simulink model "walkingRobotRL3D"  (R2020b)
settings: Solver=ode23t  StartTime=0.0  StopTime=Tf  RelTol=1e-2  EnableMultiTasking=on
PreLoadFcn:
  | robotParametersRL
undefined symbols (not defined in the file): agent, ankleD_pitch_jointMAX, ankleD_pitch_jointMIN, ankleD_roll_jointMAX, ankleD_roll_jointMIN, ankleI_pitch_jointMAX, ankleI_pitch_jointMIN, ankleI_roll_jointMAX, ankleI_roll_jointMIN, getSampleTime, height_plane, hipD_pitch_jointMAX, hipD_pitch_jointMIN, hipD_roll_jointMAX, hipD_roll_jointMIN, hipI_pitch_jointMAX, hipI_pitch_jointMIN, hipI_roll_jointMAX, hipI_roll_jointMIN, init_angs_L, init_angs_R, init_height, joint_damping, joint_limit_damping, joint_limit_stiffness, joint_stiffness, kneeD_jointMAX, kneeD_jointMIN, kneeI_jointMAX, kneeI_jointMIN, lower_leg_I0, lower_leg_length, lower_leg_mass, lower_leg_x, lower_leg_y, muscle_nominal_length, p10_ankleD_roll, plane_x, plane_y, regulator_type, tau, Tf, torso_height, torso_length, torso_offset_x, torso_offset_z, torso_width, torso_x, torso_y, torso_z, Ts, upper_leg_I0, upper_leg_length, upper_leg_mass, upper_leg_x, upper_leg_y, v10_ankleD_pitch, v10_ankleD_roll, v10_ankleI_pitch, v10_ankleI_roll ... (+41)
libraries: sm_lib x222, simulink x183, nesl_utility x130, walkingRobotUtils x69, rllib x2
(part 24 of 24)

== matlab function walkingRobotRL3D/Walking Robot (Angle based)/Antagonistic PAM Left Leg/ankleI_roll PAM/Proportional Regulator (Muscles 1) ==
  data: V1 input; reg_type input; p1 output
% Author: Eduardo Reyero Ibáñez
% Descrition: In this file it will be implemented the required input for the PAM
function p1  = propReg(V1,reg_type)
%% Proportional pressure regulators VPPM
%Range of Voltage
minVoltage = 0;
maxVoltage = 7.98; % This voltage provide 8 bar of pressure with regulator type 1
p1 = zeros(1,1);
%Select regulartor type
%reg_type = 1; % This will be given by the call of the function
%Limit the voltage
for i=1:length(p1)
if V1(i) >= maxVoltage 
    V1(i) = maxVoltage;
end
end
if reg_type == 1
    f_prop = @(V) 0.99*V+0.1;
    for i=1:length(p1)
    p1(i) = f_prop(V1(i));
    end
elseif reg_type == 2
    f_prop = @(V) 0.594*V+0.06;
    for i=1:length(p1)
    p1(i) = f_prop(V1(i));
    end
else
    f_prop = @(V) 0.198*V+0.02;
    for i=1:length(p1)
    p1(i) = f_prop(V1(i));
    end
end

% figure
% fplot(p1)
% xlim([0 10])
% ylim([0 10])
end

== matlab function walkingRobotRL3D/Walking Robot (Angle based)/Antagonistic PAM Left Leg/ankleI_roll PAM/Proportional Regulator (Muscles 2) ==
  data: V1 input; reg_type input; p1 output
% Author: Eduardo Reyero Ibáñez
% Descrition: In this file it will be implemented the required input for the PAM
function p1  = propReg(V1,reg_type)
%% Proportional pressure regulators VPPM
%Range of Voltage
minVoltage = 0;
maxVoltage = 7.98; % This voltage provide 8 bar of pressure with regulator type 1
p1 = zeros(1,1);
%Select regulartor type
%reg_type = 1; % This will be given by the call of the function
%Limit the voltage
for i=1:length(p1)
if V1(i) >= maxVoltage 
    V1(i) = maxVoltage;
end
end
if reg_type == 1
    f_prop = @(V) 0.99*V+0.1;
    for i=1:length(p1)
    p1(i) = f_prop(V1(i));
    end
elseif reg_type == 2
    f_prop = @(V) 0.594*V+0.06;
    for i=1:length(p1)
    p1(i) = f_prop(V1(i));
    end
else
    f_prop = @(V) 0.198*V+0.02;
    for i=1:length(p1)
    p1(i) = f_prop(V1(i));
    end
end

% figure
% fplot(p1)
% xlim([0 10])
% ylim([0 10])
end

== matlab function walkingRobotRL3D/Walking Robot (Angle based)/Antagonistic PAM Left Leg/ankleI_roll PAM/Spring and damping model/Stimation of spring coefficients ==
  data: P1 input; S1 output; Fload input; dmax1 input; F1 input; dmax1_per input
%Author: Eduardo Reyero
%Description: Calculate spring coefficient

function S1 = calculateSpringCoeff(P1,Fload,dmax1,F1,dmax1_per)
S1=zeros(length(dmax1),1);
%curve1 = @(x,P)  -0.002697-93.8*x+2.917*P+13.05*x^2-0.04264*x*P-0.001793*P^2-0.9395*x^3-0.001597*x^2*P-0.0001142*x*P^2+4.694e-06*P^3+0.03335*x^4+6.106e-06*x^3*P+2.699e-06*x^2*P^2+1.25e-07*x*P^3-5.675e-09*P^4-0.0004611*x^5+9.334e-07*x^4*P-1.221e-08*x^3*P^2-1.463e-09*x^2*P^3-4.929e-11*x*P^4+2.492e-12*P^5;
%F1 = zeros(length(P1),1);
for i=1:length(P1)
 %   F1(i) = curve1(dmax1_per(i),P1(i)); %Should be 0 (or aprox 0)
    S1(i) = (F1(i)-Fload(i))/dmax1(i); 
end
 
 %   S1(i) = 4379.43006090932;
end

== matlab function walkingRobotRL3D/Walking Robot (Angle based)/Antagonistic PAM Left Leg/ankleI_roll PAM/Spring and damping model/Stimation of spring coefficients1 ==
  data: F2 input; P2 input; S2 output; Fload input; dmax2 input; dmax2_per input
%Author: Eduardo Reyero
%Description: Calculate spring coefficient

function S2 = calculateSpringCoeff(F2,P2,Fload,dmax2,dmax2_per)
S2=zeros(length(dmax2),1);
%curve1 = @(x,P)  -0.002697-93.8*x+2.917*P+13.05*x^2-0.04264*x*P-0.001793*P^2-0.9395*x^3-0.001597*x^2*P-0.0001142*x*P^2+4.694e-06*P^3+0.03335*x^4+6.106e-06*x^3*P+2.699e-06*x^2*P^2+1.25e-07*x*P^3-5.675e-09*P^4-0.0004611*x^5+9.334e-07*x^4*P-1.221e-08*x^3*P^2-1.463e-09*x^2*P^3-4.929e-11*x*P^4+2.492e-12*P^5;
%F2 = zeros(length(P2),1);
for i=1:length(P2)
   % F2(i) = curve1(dmax2_per(i),P2(i)); %Should be aprox 0
    S2(i) = (F2(i)-Fload(i))/dmax2(i); 
end
  %  S2(i) = -8268.02654048148;
end

== matlab function walkingRobotRL3D/Walking Robot (Angle based)/Antagonistic PAM Left Leg/ankleI_roll PAM/Spring and damping model/getDeltaXmax/getMaxStroke1 ==
  data: P1 input; x_max1 output
%Author: Eduardo Reyero Ibáñez
%Description: Functions for obtaining the maximun stroke value of a given
%curve F(x). It is reached for the x value which makes F = 0
function x_max1 = getMaxStroke(P1)
x_range = (-3:0.01:29)'; %This range convers the %contraction for all the pressures from 0 to 8 bar
%load('StaticFxPmodel\fxpSurface.mat');

curve1 = @(x,P)  -0.002697-93.8*x+2.917*P+13.05*x^2-0.04264*x*P-0.001793*P^2-0.9395*x^3-0.001597*x^2*P-0.0001142*x*P^2+4.694e-06*P^3+0.03335*x^4+6.106e-06*x^3*P+2.699e-06*x^2*P^2+1.25e-07*x*P^3-5.675e-09*P^4-0.0004611*x^5+9.334e-07*x^4*P-1.221e-08*x^3*P^2-1.463e-09*x^2*P^3-4.929e-11*x*P^4+2.492e-12*P^5;
F_x = zeros(length(x_range),1);
for i=1:length(x_range)
    F_x(i) = curve1(x_range(i),P1);
    if F_x(i)<0
       %We have found the x axis cross
       x_max1 = x_range(i-1);
       break;
   else
        x_max1 = x_range(i); %Will never end here but need to avoid simulink error
    end
end

end

== matlab function walkingRobotRL3D/Walking Robot (Angle based)/Antagonistic PAM Left Leg/ankleI_roll PAM/Spring and damping model/getDeltaXmax1/getMaxStroke1 ==
  data: P2 input; x_max1 output
%Author: Eduardo Reyero Ibáñez
%Description: Functions for obtaining the maximun stroke value of a given
%curve F(x). It is reached for the x value which makes F = 0
function x_max1 = getMaxStroke(P2)
x_range = (-3:0.01:29)'; %This range convers the %contraction for all the pressures from 0 to 8 bar
%load('StaticFxPmodel\fxpSurface.mat');

curve1 = @(x,P)  -0.002697-93.8*x+2.917*P+13.05*x^2-0.04264*x*P-0.001793*P^2-0.9395*x^3-0.001597*x^2*P-0.0001142*x*P^2+4.694e-06*P^3+0.03335*x^4+6.106e-06*x^3*P+2.699e-06*x^2*P^2+1.25e-07*x*P^3-5.675e-09*P^4-0.0004611*x^5+9.334e-07*x^4*P-1.221e-08*x^3*P^2-1.463e-09*x^2*P^3-4.929e-11*x*P^4+2.492e-12*P^5;
F_x = zeros(length(x_range),1);
for i=1:length(x_range)
    F_x(i) = curve1(x_range(i),P2);
    if F_x(i)<0
       %We have found the x axis cross
       x_max1 = x_range(i-1);
       break;
   else
        x_max1 = x_range(i); %Will never end here but need to avoid simulink error
    end
end

end

== matlab function walkingRobotRL3D/Walking Robot1/Dynamic model of antagonistic PAM actuators/Spring//Damping (Muscles 1)/Getxmax1/getMaxStroke9 ==
  data: P1 input; x_max1 output
%Author: Eduardo Reyero Ibáñez
%Description: Functions for obtaining the maximun stroke value of a given
%curve F(x). It is reached for the x value which makes F = 0
function x_max1 = getMaxStroke(P1)
x_range = (-3:0.01:29)'; %This range convers the %contraction for all the pressures from 0 to 8 bar
%load('StaticFxPmodel\fxpSurface.mat');
curve1 = @(x,P)  -0.002697-93.8*x+2.917*P+13.05*x^2-0.04264*x*P-0.001793*P^2-0.9395*x^3-0.001597*x^2*P-0.0001142*x*P^2+4.694e-06*P^3+0.03335*x^4+6.106e-06*x^3*P+2.699e-06*x^2*P^2+1.25e-07*x*P^3-5.675e-09*P^4-0.0004611*x^5+9.334e-07*x^4*P-1.221e-08*x^3*P^2-1.463e-09*x^2*P^3-4.929e-11*x*P^4+2.492e-12*P^5;
F_x = zeros(length(x_range),1);
for i=1:length(x_range)
    F_x(i) = curve1(x_range(i),P1);
    if F_x(i)<0
       %We have found the x axis cross
       x_max1 = x_range(i-1);
       break;
   else
        x_max1 = x_range(i); %Will never end here but need to avoid simulink error
    end
end

end

== matlab function walkingRobotRL3D/Walking Robot (Angle based)/Antagonistic PAM Left Leg/ankleI_pitch PAM/F(x,P) mode (Muscles 1) ==
  data: P1 input; F1 output; x_muscle1 input
%Author: Eduardo Reyero Ibáñez
%Note: F(x) curves for different pressures are limited by recommended
%limitation of 20% in contraction percentage for the used PAM actuator
%(L = 260mm D=20mm)
function F1 = FxPmodel(P1,x_muscle1)
%Input: P comming from proporcional controller  is in bar. Its 6x1 vector
% x_muscle (in % contraction)
%Output:F according to P input and and x value of half of the maximun
%permissible stroke
%Importing 2 variable F(x,P) model
curve = @(x,P)  -0.002697-93.8*x+2.917*P+13.05*x^2-0.04264*x*P-0.001793*P^2-0.9395*x^3-0.001597*x^2*P-0.0001142*x*P^2+4.694e-06*P^3+0.03335*x^4+6.106e-06*x^3*P+2.699e-06*x^2*P^2+1.25e-07*x*P^3-5.675e-09*P^4-0.0004611*x^5+9.334e-07*x^4*P-1.221e-08*x^3*P^2-1.463e-09*x^2*P^3-4.929e-11*x*P^4+2.492e-12*P^5;
%Defining F and x vectors for the 6 actuators
F1 = zeros(length(P1),1); %6x1
x1 = zeros(length(P1),1); %6x1
% Transform P from bar to Kpa
P1 = 100*P1;

for i=1:length(P1)
% Obtaining the stroke
x1(i) = x_muscle1(i); 
% Obtaining the applied force
F1(i) = curve(x1(i),P1(i)); 
% if F1(i)<0
%     F1(i) = 0;
% end
end
end

== matlab function walkingRobotRL3D/Walking Robot (Angle based)/Antagonistic PAM Left Leg/ankleI_pitch PAM/F(x,P) mode (Muscles 1)1 ==
  data: P2 input; F2 output; x_muscle2 input
%Author: Eduardo Reyero Ibáñez
%Note: F(x) curves for different pressures are limited by recommended
%limitation of 20% in contraction percentage for the used PAM actuator
%(L = 260mm D=20mm)
function F2 = FxPmodel(P2,x_muscle2)
%Input: P comming from proporcional controller  is in bar. Its 6x1 vector
% x_muscle (in % contraction)
%Output:F according to P input and and x value of half of the maximun
%permissible stroke
%Importing 2 variable F(x,P) model
curve = @(x,P)  -0.002697-93.8*x+2.917*P+13.05*x^2-0.04264*x*P-0.001793*P^2-0.9395*x^3-0.001597*x^2*P-0.0001142*x*P^2+4.694e-06*P^3+0.03335*x^4+6.106e-06*x^3*P+2.699e-06*x^2*P^2+1.25e-07*x*P^3-5.675e-09*P^4-0.0004611*x^5+9.334e-07*x^4*P-1.221e-08*x^3*P^2-1.463e-09*x^2*P^3-4.929e-11*x*P^4+2.492e-12*P^5;
%Defining F and x vectors for the 6 actuators
F2 = zeros(length(P2),1); %6x1
x2 = zeros(length(P2),1); %6x1
% Transform P from bar to Kpa
P2 = 100*P2;

for i=1:length(P2)
% Obtaining the stroke
x2(i) = x_muscle2(i); 
% Obtaining the applied force
F2(i) = curve(x2(i),P2(i));
% if F2(i)<0
%     F2(i) = 0;
% end
end
end

== matlab function walkingRobotRL3D/Walking Robot (Angle based)/Antagonistic PAM Left Leg/ankleI_pitch PAM/Proportional Regulator (Muscles 1) ==
  data: V1 input; reg_type input; p1 output
% Author: Eduardo Reyero Ibáñez
% Descrition: In this file it will be implemented the required input for the PAM
function p1  = propReg(V1,reg_type)
%% Proportional pressure regulators VPPM
%Range of Voltage
minVoltage = 0;
maxVoltage = 7.98; % This voltage provide 8 bar of pressure with regulator type 1
p1 = zeros(1,1);
%Select regulartor type
%reg_type = 1; % This will be given by the call of the function
%Limit the voltage
for i=1:length(p1)
if V1(i) >= maxVoltage 
    V1(i) = maxVoltage;
end
end
if reg_type == 1
    f_prop = @(V) 0.99*V+0.1;
    for i=1:length(p1)
    p1(i) = f_prop(V1(i));
    end
elseif reg_type == 2
    f_prop = @(V) 0.594*V+0.06;
    for i=1:length(p1)
    p1(i) = f_prop(V1(i));
    end
else
    f_prop = @(V) 0.198*V+0.02;
    for i=1:length(p1)
    p1(i) = f_prop(V1(i));
    end
end

% figure
% fplot(p1)
% xlim([0 10])
% ylim([0 10])
end

== matlab function walkingRobotRL3D/Walking Robot (Angle based)/Antagonistic PAM Left Leg/ankleI_pitch PAM/Proportional Regulator (Muscles 2) ==
  data: V1 input; reg_type input; p1 output
% Author: Eduardo Reyero Ibáñez
% Descrition: In this file it will be implemented the required input for the PAM
function p1  = propReg(V1,reg_type)
%% Proportional pressure regulators VPPM
%Range of Voltage
minVoltage = 0;
maxVoltage = 7.98; % This voltage provide 8 bar of pressure with regulator type 1
p1 = zeros(1,1);
%Select regulartor type
%reg_type = 1; % This will be given by the call of the function
%Limit the voltage
for i=1:length(p1)
if V1(i) >= maxVoltage 
    V1(i) = maxVoltage;
end
end
if reg_type == 1
    f_prop = @(V) 0.99*V+0.1;
    for i=1:length(p1)
    p1(i) = f_prop(V1(i));
    end
elseif reg_type == 2
    f_prop = @(V) 0.594*V+0.06;
    for i=1:length(p1)
    p1(i) = f_prop(V1(i));
    end
else
    f_prop = @(V) 0.198*V+0.02;
    for i=1:length(p1)
    p1(i) = f_prop(V1(i));
    end
end

% figure
% fplot(p1)
% xlim([0 10])
% ylim([0 10])
end

== matlab function walkingRobotRL3D/Walking Robot (Angle based)/Antagonistic PAM Left Leg/ankleI_pitch PAM/Spring and damping model/Stimation of spring coefficients ==
  data: P1 input; S1 output; Fload input; dmax1 input; F1 input; dmax1_per input
%Author: Eduardo Reyero
%Description: Calculate spring coefficient

function S1 = calculateSpringCoeff(P1,Fload,dmax1,F1,dmax1_per)
S1=zeros(length(dmax1),1);
%curve1 = @(x,P)  -0.002697-93.8*x+2.917*P+13.05*x^2-0.04264*x*P-0.001793*P^2-0.9395*x^3-0.001597*x^2*P-0.0001142*x*P^2+4.694e-06*P^3+0.03335*x^4+6.106e-06*x^3*P+2.699e-06*x^2*P^2+1.25e-07*x*P^3-5.675e-09*P^4-0.0004611*x^5+9.334e-07*x^4*P-1.221e-08*x^3*P^2-1.463e-09*x^2*P^3-4.929e-11*x*P^4+2.492e-12*P^5;
%F1 = zeros(length(P1),1);
for i=1:length(P1)
 %   F1(i) = curve1(dmax1_per(i),P1(i)); %Should be 0 (or aprox 0)
    S1(i) = (F1(i)-Fload(i))/dmax1(i); 
end
 
 %   S1(i) = 4379.43006090932;
end

== matlab function walkingRobotRL3D/Walking Robot (Angle based)/Antagonistic PAM Left Leg/ankleI_pitch PAM/Spring and damping model/Stimation of spring coefficients1 ==
  data: F2 input; P2 input; S2 output; Fload input; dmax2 input; dmax2_per input
%Author: Eduardo Reyero
%Description: Calculate spring coefficient

function S2 = calculateSpringCoeff(F2,P2,Fload,dmax2,dmax2_per)
S2=zeros(length(dmax2),1);
%curve1 = @(x,P)  -0.002697-93.8*x+2.917*P+13.05*x^2-0.04264*x*P-0.001793*P^2-0.9395*x^3-0.001597*x^2*P-0.0001142*x*P^2+4.694e-06*P^3+0.03335*x^4+6.106e-06*x^3*P+2.699e-06*x^2*P^2+1.25e-07*x*P^3-5.675e-09*P^4-0.0004611*x^5+9.334e-07*x^4*P-1.221e-08*x^3*P^2-1.463e-09*x^2*P^3-4.929e-11*x*P^4+2.492e-12*P^5;
%F2 = zeros(length(P2),1);
for i=1:length(P2)
   % F2(i) = curve1(dmax2_per(i),P2(i)); %Should be aprox 0
    S2(i) = (F2(i)-Fload(i))/dmax2(i); 
end
  %  S2(i) = -8268.02654048148;
end

== matlab function walkingRobotRL3D/Walking Robot (Angle based)/Antagonistic PAM Left Leg/ankleI_pitch PAM/Spring and damping model/getDeltaXmax/getMaxStroke1 ==
  data: P1 input; x_max1 output
%Author: Eduardo Reyero Ibáñez
%Description: Functions for obtaining the maximun stroke value of a given
%curve F(x). It is reached for the x value which makes F = 0
function x_max1 = getMaxStroke(P1)
x_range = (-3:0.01:29)'; %This range convers the %contraction for all the pressures from 0 to 8 bar
%load('StaticFxPmodel\fxpSurface.mat');

curve1 = @(x,P)  -0.002697-93.8*x+2.917*P+13.05*x^2-0.04264*x*P-0.001793*P^2-0.9395*x^3-0.001597*x^2*P-0.0001142*x*P^2+4.694e-06*P^3+0.03335*x^4+6.106e-06*x^3*P+2.699e-06*x^2*P^2+1.25e-07*x*P^3-5.675e-09*P^4-0.0004611*x^5+9.334e-07*x^4*P-1.221e-08*x^3*P^2-1.463e-09*x^2*P^3-4.929e-11*x*P^4+2.492e-12*P^5;
F_x = zeros(length(x_range),1);
for i=1:length(x_range)
    F_x(i) = curve1(x_range(i),P1);
    if F_x(i)<0
       %We have found the x axis cross
       x_max1 = x_range(i-1);
       break;
   else
        x_max1 = x_range(i); %Will never end here but need to avoid simulink error
    end
end

end

== matlab function walkingRobotRL3D/Walking Robot (Angle based)/Antagonistic PAM Left Leg/ankleI_pitch PAM/Spring and damping model/getDeltaXmax1/getMaxStroke1 ==
  data: P2 input; x_max1 output
%Author: Eduardo Reyero Ibáñez
%Description: Functions for obtaining the maximun stroke value of a given
%curve F(x). It is reached for the x value which makes F = 0
function x_max1 = getMaxStroke(P2)
x_range = (-3:0.01:29)'; %This range convers the %contraction for all the pressures from 0 to 8 bar
%load('StaticFxPmodel\fxpSurface.mat');

curve1 = @(x,P)  -0.002697-93.8*x+2.917*P+13.05*x^2-0.04264*x*P-0.001793*P^2-0.9395*x^3-0.001597*x^2*P-0.0001142*x*P^2+4.694e-06*P^3+0.03335*x^4+6.106e-06*x^3*P+2.699e-06*x^2*P^2+1.25e-07*x*P^3-5.675e-09*P^4-0.0004611*x^5+9.334e-07*x^4*P-1.221e-08*x^3*P^2-1.463e-09*x^2*P^3-4.929e-11*x*P^4+2.492e-12*P^5;
F_x = zeros(length(x_range),1);
for i=1:length(x_range)
    F_x(i) = curve1(x_range(i),P2);
    if F_x(i)<0
       %We have found the x axis cross
       x_max1 = x_range(i-1);
       break;
   else
        x_max1 = x_range(i); %Will never end here but need to avoid simulink error
    end
end

end

== matlab function walkingRobotRL3D/Walking Robot (Angle based)/Antagonistic PAM Left Leg/hipI_pitch PAM/F(x,P) mode (Muscles 1) ==
  data: P1 input; F1 output; x_muscle1 input
%Author: Eduardo Reyero Ibáñez
%Note: F(x) curves for different pressures are limited by recommended
%limitation of 20% in contraction percentage for the used PAM actuator
%(L = 260mm D=20mm)
function F1 = FxPmodel(P1,x_muscle1)
%Input: P comming from proporcional controller  is in bar. Its 6x1 vector
% x_muscle (in % contraction)
%Output:F according to P input and and x value of half of the maximun
%permissible stroke
%Importing 2 variable F(x,P) model
curve = @(x,P)  -0.002697-93.8*x+2.917*P+13.05*x^2-0.04264*x*P-0.001793*P^2-0.9395*x^3-0.001597*x^2*P-0.0001142*x*P^2+4.694e-06*P^3+0.03335*x^4+6.106e-06*x^3*P+2.699e-06*x^2*P^2+1.25e-07*x*P^3-5.675e-09*P^4-0.0004611*x^5+9.334e-07*x^4*P-1.221e-08*x^3*P^2-1.463e-09*x^2*P^3-4.929e-11*x*P^4+2.492e-12*P^5;
%Defining F and x vectors for the 6 actuators
F1 = zeros(length(P1),1); %6x1
x1 = zeros(length(P1),1); %6x1
% Transform P from bar to Kpa
P1 = 100*P1;

for i=1:length(P1)
% Obtaining the stroke
x1(i) = x_muscle1(i); 
% Obtaining the applied force
F1(i) = curve(x1(i),P1(i)); 
% if F1(i)<0
%     F1(i) = 0;
% end
end
end

== matlab function walkingRobotRL3D/Walking Robot1/Dynamic model of antagonistic PAM actuators/Spring//Damping (Muscles 1)/Getxmax1/getMaxStroke ==
  data: P1 input; x_max1 output
%Author: Eduardo Reyero Ibáñez
%Description: Functions for obtaining the maximun stroke value of a given
%curve F(x). It is reached for the x value which makes F = 0
function x_max1 = getMaxStroke(P1)
x_range = (-3:0.01:29)'; %This range convers the %contraction for all the pressures from 0 to 8 bar
%load('StaticFxPmodel\fxpSurface.mat');
curve1 = @(x,P)  -0.002697-93.8*x+2.917*P+13.05*x^2-0.04264*x*P-0.001793*P^2-0.9395*x^3-0.001597*x^2*P-0.0001142*x*P^2+4.694e-06*P^3+0.03335*x^4+6.106e-06*x^3*P+2.699e-06*x^2*P^2+1.25e-07*x*P^3-5.675e-09*P^4-0.0004611*x^5+9.334e-07*x^4*P-1.221e-08*x^3*P^2-1.463e-09*x^2*P^3-4.929e-11*x*P^4+2.492e-12*P^5;
F_x = zeros(length(x_range),1);
for i=1:length(x_range)
    F_x(i) = curve1(x_range(i),P1);
    if F_x(i)<0
       %We have found the x axis cross
       x_max1 = x_range(i-1);
       break;
   else
        x_max1 = x_range(i); %Will never end here but need to avoid simulink error
    end
end

end

== matlab function walkingRobotRL3D/Walking Robot (Angle based)/Antagonistic PAM Left Leg/hipI_pitch PAM/F(x,P) mode (Muscles 1)1 ==
  data: P2 input; F2 output; x_muscle2 input
%Author: Eduardo Reyero Ibáñez
%Note: F(x) curves for different pressures are limited by recommended
%limitation of 20% in contraction percentage for the used PAM actuator
%(L = 260mm D=20mm)
function F2 = FxPmodel(P2,x_muscle2)
%Input: P comming from proporcional controller  is in bar. Its 6x1 vector
% x_muscle (in % contraction)
%Output:F according to P input and and x value of half of the maximun
%permissible stroke
%Importing 2 variable F(x,P) model
curve = @(x,P)  -0.002697-93.8*x+2.917*P+13.05*x^2-0.04264*x*P-0.001793*P^2-0.9395*x^3-0.001597*x^2*P-0.0001142*x*P^2+4.694e-06*P^3+0.03335*x^4+6.106e-06*x^3*P+2.699e-06*x^2*P^2+1.25e-07*x*P^3-5.675e-09*P^4-0.0004611*x^5+9.334e-07*x^4*P-1.221e-08*x^3*P^2-1.463e-09*x^2*P^3-4.929e-11*x*P^4+2.492e-12*P^5;
%Defining F and x vectors for the 6 actuators
F2 = zeros(length(P2),1); %6x1
x2 = zeros(length(P2),1); %6x1
% Transform P from bar to Kpa
P2 = 100*P2;

for i=1:length(P2)
% Obtaining the stroke
x2(i) = x_muscle2(i); 
% Obtaining the applied force
F2(i) = curve(x2(i),P2(i));
% if F2(i)<0
%     F2(i) = 0;
% end
end
end
